simulink model "EPRModel"  (R2022a)
settings: Solver=ode5  StartTime=0.0  StopTime=inf  RelTol=1e-3
InitFcn:
  | eprecorder_mdl_init_callback();
StopFcn:
  | eprecorder_mdl_stop_callback;
undefined symbols (not defined in the file or in its folder): EPR, eprecorder_online_on_triggered, eprecorder_online_on_viewer_triggered
libraries: simulink x3, sldrtlib x1
settings Model: Creator=Neurolab  LastModifiedBy=bo11r
settings SolverCC: AlgebraicLoopSolver=TrustRegion
settings DebuggingCC: UnconnectedInputMsg=warning  UnconnectedOutputMsg=warning  UnconnectedLineMsg=warning  SFMachineParentedDataDiag=warning
settings RTWCC: Description=Simulink Desktop Real-Time  SystemTargetFile=sldrt.tlc  TemplateMakefile=sldrt.tmf  RTWCompilerOptimization=on  DLArmComputeVersion=19.05
settings CodeAppCC: MaxIdLength=95
settings SimulinkDesktopRealTimeCC: TargetPreCompLibLocation=C:\Program Files\MATLAB\R2020b\toolbox\sldrt\lib\win64

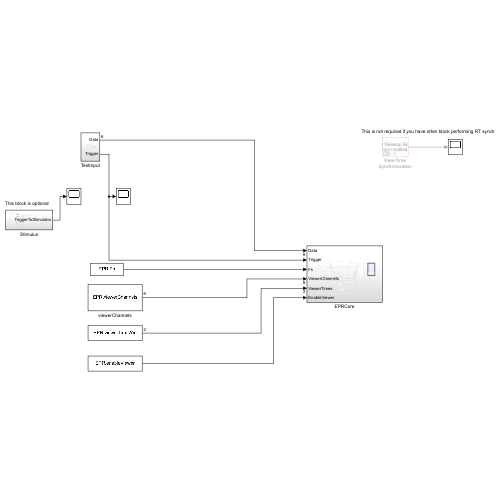
[thumbnail: Simulink's stored preview of the top-level diagram]
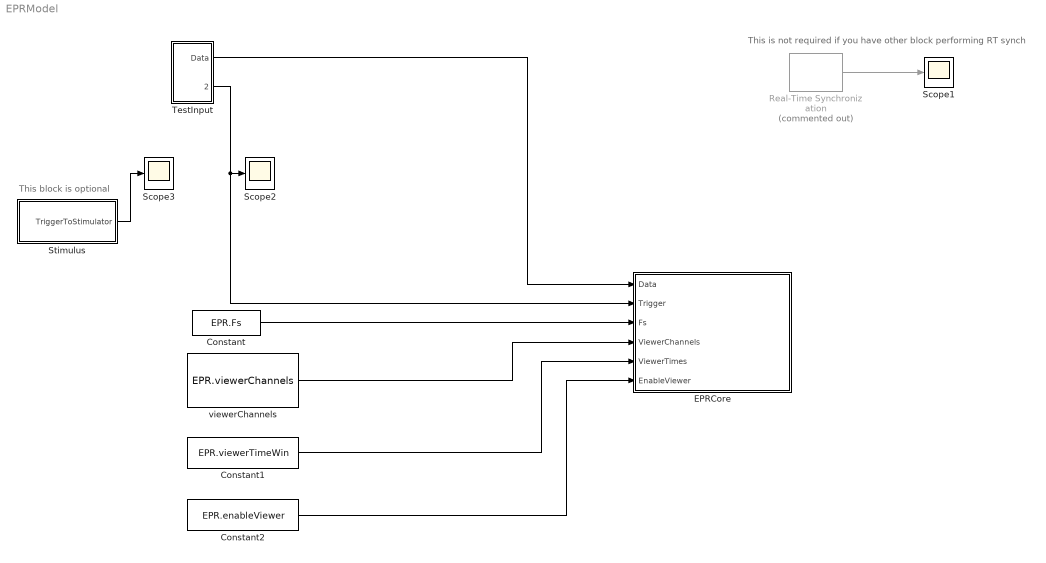
== system EPRModel ==
  note: This block is optional
  note: This is not required if you have other block performing RT synch
  Constant : Constant  Value=EPR.Fs
  Constant1 : Constant  Value=EPR.viewerTimeWin
  Constant2 : Constant  Value=EPR.enableViewer
  EPRCore : Subsystem
  Real-Time Synchronization : sldrtlib/Real-Time Synchronization  Commented=on  SampleTime=1/EPR.Fs  MaxMissedTicks=1000  ShowMissedTicks=on  YieldWhenWaiting=off
  Scope1 : Scope
  Scope2 : Scope
  Scope3 : Scope
  Stimulus : Subsystem
  TestInput : Subsystem
  viewerChannels : Constant  Value=EPR.viewerChannels  mask(Creates axes for plottint EP){}
      mask init:
      | %{
      |  p=[403   246   560   420]
      |  u='pixels'
      | if(length(findobj('tag','EMG000')))
      |      h=figure(findobj('tag','EMG000'));
      |      p=get(h,'position');
      |      u=get(h,'units');
      |      close(h);
      | end
      |      figure1 = figure('numbertitle','off','name','EP','tag','EMG000');
      |      set(figure1,'units',u);
      |      set(figure1,'position',p);
      |      % Create axes
      |      MYEP.axes(1)=subplot(3,1,1);
      |       title('Channels 1 avg')
      |       box(MYEP.axes(1),'on');
      |       hold(MYEP.axes(1),'all');
      | 
      |      MYEP.axes(2)=subplot(3,1,2);
      |       title('Channels 2 avg')
      |       box(MYEP.axes(2),'on');
      |       hold(MYEP.axes(2),'all');
      | 
      |      MYEP.axes(3)=subplot(3,1,3);
      |      title('Channels 3 avg')
      |      xlabel('1 sec Samples since stimulus onset')
      |      ylabel('Avg amplitude (micro volts)')
      |      box(MYEP.axes(3),'on');
      |      hold(MYEP.axes(3),'all');
      | 
      | %}
  wires:
  viewerChannels/1 -> EPRCore/4(ViewerChannels)
  Constant/1 -> EPRCore/3(Fs)
  Constant1/1 -> EPRCore/5(ViewerTimes)
  Constant2/1 -> EPRCore/6(EnableViewer)
  Real-Time Synchronization/1 -> Scope1/1
  TestInput/1(Data) -> EPRCore/1(Data)
  TestInput/2(Trigger) -> EPRCore/2(Trigger), Scope2/1
  Stimulus/1(TriggerToStimulator) -> Scope3/1

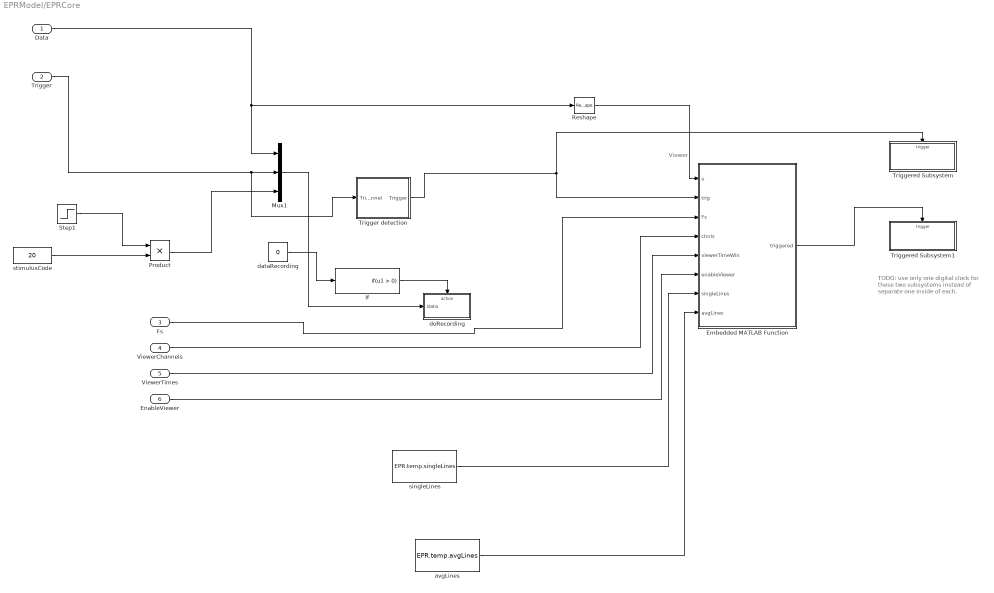
== system EPRModel/EPRCore ==
  note: TODO: use only one digital clock
      | for these two subsystems instead
      | of separate one inside of each.
  note: Viewer
  Data : Inport
  Trigger : Inport  Port=2
  Fs : Inport  Port=3
  ViewerChannels : Inport  Port=4
  ViewerTimes : Inport  Port=5
  EnableViewer : Inport  Port=6
  Embedded MATLAB Function : MATLAB Function  TreatAsAtomicUnit=on
  If : If  ShowElse=off
  Mux1 : Mux  Inputs=3
  Product : Product
  Reshape : Reshape
  Step1 : Step  Before=1  SampleTime=0
  Trigger detection : Subsystem
  Triggered Subsystem : Subsystem  TreatAsAtomicUnit=on
  Triggered Subsystem1 : Subsystem  TreatAsAtomicUnit=on
  avgLines : Constant  Value=EPR.temp.avgLines  mask(Creates axes for plottint EP){}
      mask init: same as EPRModel/viewerChannels
  dataRecording : Constant  Value=0
  doRecording : Subsystem  TreatAsAtomicUnit=on
  singleLines : Constant  Value=EPR.temp.singleLines  mask(Creates axes for plottint EP){}
      mask init: same as EPRModel/viewerChannels
  stimulusCode : Constant  Value=20
  wires:
  If/1 -> doRecording/Action
  Data/1 -> Mux1/1, Reshape/1
  dataRecording/1 -> If/1
  ViewerChannels/1 -> Embedded MATLAB Function/4(chnls)
  Trigger/1 -> Trigger detection/1(Trigger channel), Mux1/2
  Mux1/1 -> doRecording/1(data)
  Fs/1 -> Embedded MATLAB Function/3(Fs)
  ViewerTimes/1 -> Embedded MATLAB Function/5(viewerTimeWin)
  EnableViewer/1 -> Embedded MATLAB Function/6(enableViewer)
  Reshape/1 -> Embedded MATLAB Function/1(u)
  stimulusCode/1 -> Product/2
  Step1/1 -> Product/1
  Product/1 -> Mux1/3
  singleLines/1 -> Embedded MATLAB Function/7(singleLines)
  avgLines/1 -> Embedded MATLAB Function/8(avgLines)
  Embedded MATLAB Function/1(triggered) -> Triggered Subsystem1/Trigger
  Trigger detection/1(Trigger) -> Embedded MATLAB Function/2(trig), Triggered Subsystem/Trigger

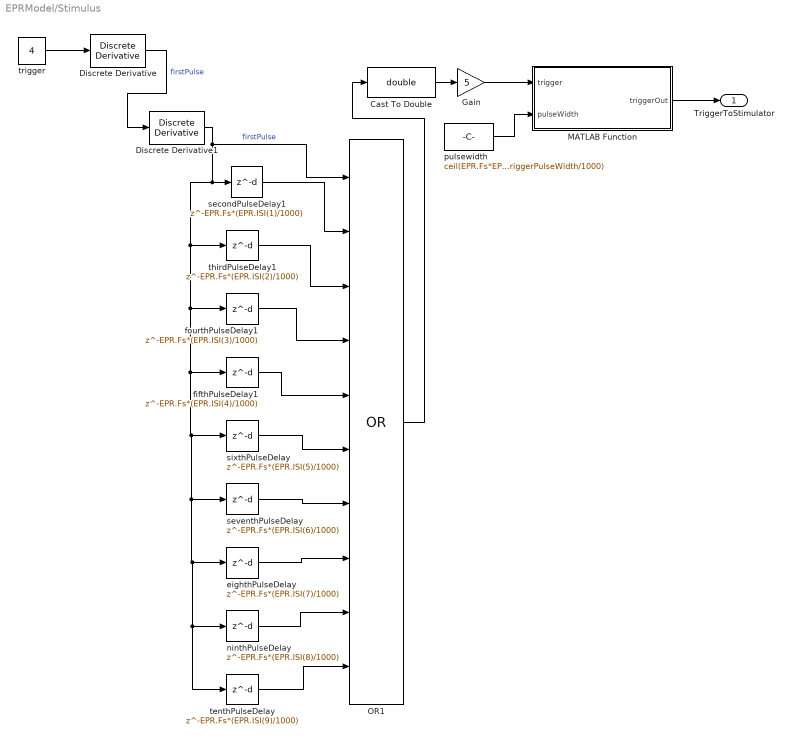
== system EPRModel/Stimulus ==
  Cast To Double : DataTypeConversion  OutDataTypeStr=double  SaturateOnIntegerOverflow=off  RndMeth=Floor
  Discrete Derivative : simulink/Discrete/Discrete Derivative  gainval=1.0  ICPrevScaledInput=0.0  OutMin=[]  OutMax=[]  OutDataType=fixdt(1, 16)  OutScaling=2^-10  DoSatur=off
  Discrete Derivative1 : simulink/Discrete/Discrete Derivative  gainval=1.0  ICPrevScaledInput=0.0  OutMin=[]  OutMax=[]  OutDataType=fixdt(1, 16)  OutScaling=2^-10  DoSatur=off
  Gain : Gain  Gain=5
  MATLAB Function : MATLAB Function  TreatAsAtomicUnit=on
  OR1 : Logic  Operator=OR  Inputs=10  IconShape=distinctive  AllPortsSameDT=off  OutDataTypeStr=boolean
  eighthPulseDelay : Delay  DelayLength=EPR.Fs*(EPR.ISI(7)/1000)
  fifthPulseDelay1 : Delay  DelayLength=EPR.Fs*(EPR.ISI(4)/1000)
  fourthPulseDelay1 : Delay  DelayLength=EPR.Fs*(EPR.ISI(3)/1000)
  ninthPulseDelay : Delay  DelayLength=EPR.Fs*(EPR.ISI(8)/1000)
  pulsewidth : Constant  Value=ceil(EPR.Fs*EPR.stimulusTriggerPulseWidth/1000)
  secondPulseDelay1 : Delay  DelayLength=EPR.Fs*(EPR.ISI(1)/1000)
  seventhPulseDelay : Delay  DelayLength=EPR.Fs*(EPR.ISI(6)/1000)
  sixthPulseDelay : Delay  DelayLength=EPR.Fs*(EPR.ISI(5)/1000)
  tenthPulseDelay : Delay  DelayLength=EPR.Fs*(EPR.ISI(9)/1000)
  thirdPulseDelay1 : Delay  DelayLength=EPR.Fs*(EPR.ISI(2)/1000)
  trigger : Constant  Value=4
  TriggerToStimulator : Outport
  wires:
  OR1/1 -> Cast To Double/1
  trigger/1 -> Discrete Derivative/1
  Cast To Double/1 -> Gain/1
  Gain/1 -> MATLAB Function/1(trigger)
  pulsewidth/1 -> MATLAB Function/2(pulseWidth)
  MATLAB Function/1(triggerOut) -> TriggerToStimulator/1
  tenthPulseDelay/1 -> OR1/10
  eighthPulseDelay/1 -> OR1/8
  seventhPulseDelay/1 -> OR1/7
  ninthPulseDelay/1 -> OR1/9
  thirdPulseDelay1/1 -> OR1/3
  Discrete Derivative1/1 -> tenthPulseDelay/1, ninthPulseDelay/1, eighthPulseDelay/1, seventhPulseDelay/1, sixthPulseDelay/1, fifthPulseDelay1/1, fourthPulseDelay1/1, thirdPulseDelay1/1, secondPulseDelay1/1, OR1/1  "firstPulse"
  fifthPulseDelay1/1 -> OR1/5
  sixthPulseDelay/1 -> OR1/6
  fourthPulseDelay1/1 -> OR1/4
  secondPulseDelay1/1 -> OR1/2
  Discrete Derivative/1 -> Discrete Derivative1/1  "firstPulse"

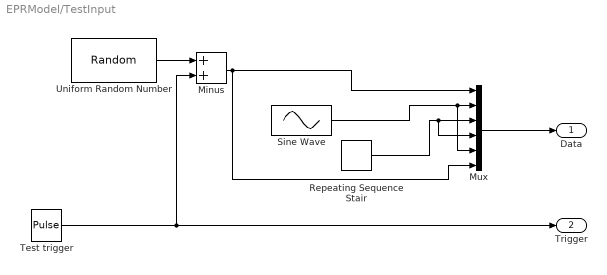
== system EPRModel/TestInput ==
  Minus : Sum
  Mux : Mux  Inputs=6
  Repeating Sequence Stair : simulink/Sources/Repeating Sequence Stair  OutValues=[3 1 4 2 1].'  tsamp=-1  OutMin=[]  OutMax=[]  OutDataTypeStr=double  OutputDataTypeScalingMode=double  OutDataType=fixdt(0,8)  ConRadixGroup=Best Precision: Vector-wise  OutScaling=2^-12
  Sine Wave : Sin  SampleTime=0
  Test trigger : DiscretePulseGenerator  Amplitude=4  Period=3*EPR.Fs  PulseWidth=max(round(0.001*EPR.Fs),1)  SampleTime=1/EPR.Fs
  Uniform Random Number : UniformRandomNumber  SampleTime=1/EPR.Fs
  Data : Outport
  Trigger : Outport  Port=2
  wires:
  Mux/1 -> Data/1
  Uniform Random Number/1 -> Minus/1
  Repeating Sequence Stair/1 -> Mux/4, Mux/3
  Sine Wave/1 -> Mux/5, Mux/2
  Test trigger/1 -> Minus/2, Trigger/1
  Minus/1 -> Mux/6, Mux/1

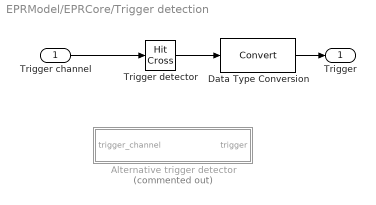
== system EPRModel/EPRCore/Trigger detection ==
  Trigger channel : Inport
  Alternative trigger detector : MATLAB Function  Commented=on  TreatAsAtomicUnit=on
  Data Type Conversion : DataTypeConversion  SaturateOnIntegerOverflow=off  RndMeth=Floor
  Trigger detector : HitCross  HitCrossingOffset=1  HitCrossingDirection=rising
  Trigger : Outport
  wires:
  Trigger detector/1 -> Data Type Conversion/1
  Trigger channel/1 -> Trigger detector/1
  Data Type Conversion/1 -> Trigger/1

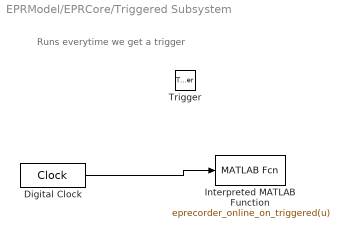
== system EPRModel/EPRCore/Triggered Subsystem ==
  note: Runs everytime we get a trigger
  Trigger : TriggerPort  TriggerTime=on sample time hit  VariantControl=(inherit)
  Digital Clock : DigitalClock  SampleTime=-1
  Interpreted MATLAB Function : MATLABFcn  MATLABFcn=eprecorder_online_on_triggered(u)  OutputDimensions=0
  wires:
  Digital Clock/1 -> Interpreted MATLAB Function/1

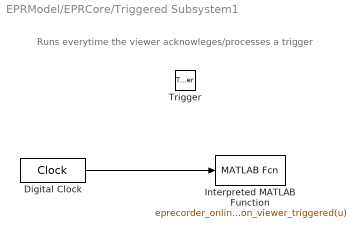
== system EPRModel/EPRCore/Triggered Subsystem1 ==
  note: Runs everytime the viewer acknowleges/processes a trigger
  Trigger : TriggerPort  TriggerTime=on sample time hit  VariantControl=(inherit)
  Digital Clock : DigitalClock  SampleTime=-1
  Interpreted MATLAB Function : MATLABFcn  MATLABFcn=eprecorder_online_on_viewer_triggered(u)  OutputDimensions=0
  wires:
  Digital Clock/1 -> Interpreted MATLAB Function/1

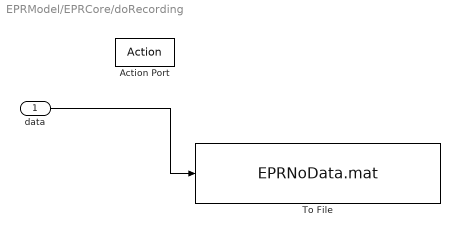
== system EPRModel/EPRCore/doRecording ==
  data : Inport
  Action Port : ActionPort  ActionPortLabel=if(u1 > 0)
  To File : ToFile  Filename=EPRNoData.mat  MatrixName=EPdata
  wires:
  data/1 -> To File/1

== matlab function EPRModel/EPRCore/Embedded MATLAB Function ==
  data: u input; trig input; Fs input; chnls input; viewerTimeWin input; enableViewer input; singleLines input; avgLines input; triggered output
function triggered=fcn(u,trig,Fs,chnls,viewerTimeWin,enableViewer,singleLines,avgLines)
%#codegen
coder.extrinsic('set');
%% EPR viewer
% [INPUT]
% u: Current data.
% trig: Trigger channel. Trigger is detected when value is 1 or greater. A
% trigger is ignored if it collides with a previous trigger. The implicit
% collision detection is based on viewerTimeWin arguement.
% Fs: Sample rate.
% chnls: the indexes of channels to display.
% viewerTimeWin: Two element vector. Where the first element is the start time
%   and the second element is end time in ms for window of data to display. 
% enableViewer: When equivalent to false, nothing will be done.
% singleLines: The main data line plot handles for each axes for non-avg
%   data where latest data will be plotted. Must correspond to chnls.
% avgAxes: The line plot handles where to display the running avg. Must
%   correspond to chnls.
% [OUTPUT]
% triggered: int<0,1> A value of 1 if trigger recieved is acknowledged or
%   processed and value of zero no trigger is recieved or trigger sent is
%   ignored because it collided with a previous trigger.
% 
persistent bufferData sumData sT numAVG tAxes recordLen;

triggered=0;

if(~enableViewer)
    return
end

if(isempty(bufferData))% init
    
    sT=-1;
    numAVG=0;%increamented at each trigger to count the number of averages
    
    % Display window sample samples
    dispWin=zeros(2,1);
    dispWin(1)=round(viewerTimeWin(1)/1000*Fs) +1;% convert to sample. We add 1 b/c matlab starts at 1 but time starts at zero
    dispWin(2)=round(viewerTimeWin(2)/1000*Fs) +1;% convert to smaple.
    tAxes=(dispWin(1)-1:dispWin(2)-1)/Fs*1000;% We subtract 1 b/c samples in matlab starts from 1 while time start from zero.
    
    % Data Buffer
    recordLen=dispWin(2); %i.e the length of data to acquire start from trigger to the end
    
    bufferLen=dispWin(2)-dispWin(1)+1;% we add 1 because to make it inclusive of the starting point, i.e dispWin(1). We can also get this as length(tAxes).
    
    % Data
    nChnls=length(chnls);%number of channels
    sumData=zeros(bufferLen,nChnls);

    bufferData=zeros(bufferLen,nChnls);
    
end

% Fifo. Append new data at the end
bufferData(1:end-1,:)=bufferData(2:end,:);
bufferData(end,:)=u(chnls)';


%collect data only at onset of stimulation if 'sT'<0 ('sT'<0 =>avoid
%collision of triggers by ignoring subsequent triggers untill 'data1' is
%filled. Actually it is better to allow the trigger to restart if trigers
%collide but this will lead to wrong number of averages. The best solution
%is not to let triggers collide. One trigger period is the onset of the
%trigger to the time the data for the trigger is collected)     
if trig(1) >=1 && sT<0 
    sT=recordLen;
    triggered=1;
end
sT=sT-1;


if sT==0
   
   sumData=sumData+bufferData;
   numAVG=numAVG+1;

   for n=1:length(chnls)
       
       %Plot last window
       if(numAVG==1)% The x-axes only need to be set once
           set(singleLines(n),'XData',tAxes);
       end
       set(singleLines(n),'YData',bufferData(:,n));
       
       
       % Plo avg
       if(numAVG==1)% The x-axes only need to be set once
           set(avgLines(n),'XData',tAxes);
       end
       set(avgLines(n),'YData',sumData(:,n)/numAVG);
   end
    
end
% all that glitter is not gold;http://www.youtube.com/watch?v=LWK4NWS479s

== matlab function EPRModel/EPRCore/Trigger detection/Alternative trigger detector ==
  data: trigger_channel input; trigger output
function trigger = fcn(trigger_channel)
% Outputs 1 when trigger_channel is at least 1, or zero otherwise.
persistent prev_trigger_channel;

thresh=1;% detection threshold

if(isempty(prev_trigger_channel))
    prev_trigger_channel=0;
end

trigger=0;
if( (trigger_channel-prev_trigger_channel) >=thresh)
    trigger=1;
end

prev_trigger_channel=trigger_channel;

== matlab function EPRModel/Stimulus/MATLAB Function ==
  data: trigger input; triggerOut output; pulseWidth input
function triggerOut = fcn(trigger,pulseWidth)
    % Hold the trigger until pulse width is reached.
    % [INPUT]
    % trigger: the value of the trigger.
    % pulseWidth: the pulse width in samples.

    persistent heldTrigger t;
    if isempty(t)
        t=0;
        heldTrigger=0;
    end

    if trigger>0
        t=pulseWidth;
        heldTrigger=trigger;
    end
    
    if(t>0)
        t=t-1;
        triggerOut=heldTrigger;
    else
        triggerOut=trigger;
    end
